simulink model "different_inverter_controls_BPS"  (R2024b)
settings: Solver=ode4  StartTime=0.0  StopTime=5  FixedStep=Ts  RelTol=1e-3
InitFcn:
  | %mode_of_operation=1;
  | %BESS_control_mode=1;
  | %Gen_Q_Control =1;
  | 
  | %Exciter_init;
  | 
  | %Exciter_init
  | Xq=0.474;
  | %%====================================================
  | % ST6C Exciter Parameters
  | 
  | KPA=30;
  | KIA=59.91;
  | KFF=1;
  | KM=1;
  | KLR=22.47;
  | KCL=1.04;
  | VAMAX=7.05;
  | VAMIN=-6.11;
  | VRMAX=7.05;
  | VRMIN=-6.11;
  | ILR=5.02;
  | KG=1;
  | TG=0.024;
  | TA=0.01;
  | VBMAX=999;
  | VMMAX=7.05;
  | VMMIN=-6.11;
  | KI=0;
  | Kp=1;
  | Kc=0;
  | Vt0=0;
  | VAAMAX=VAMAX;
  | %%========================================================
  | % UEL2C parameters
  | 
  | TUQ=.005;
  | TUP=0.050;
  | TUV=0.2;
  | TQREF=0;
  | Tadj=0;
  | K1=0;
  | K2=2;
  | VBIAS=1;
  | KFB=0;
  | TUL=0;
  | VUImax=1;
  | VUImin=-1;
  | VUELmax1=1;
  | VUELmax2=1;
  | VUELmin1=-1;
  | VUELmin2=-1;
  | KUF=0;
  | KUL=0.24;
  | KUI=0.001;
  | TU1=0;TU2=0;TU3=0;TU4=0;
  | KFIX=1;
  | VF=0;
  | VFB=0;
  | %%===========================================================
  | ... (+60 lines)
values from neighbouring files (symbols this model uses):
  inv1 = struct    [multiInverterParams.m]
  kp_sync = KQ_p/10    (= 0.04)    [multiInverterParams.m]
  Vdc = 1000    [multiInverterParams.m]
  Vpp = 480    [multiInverterParams.m]
undefined symbols (not defined in the file or in its folder): D1, Delta, DiscIntNeverNeededParam, Ion, Lithium, sigbuilder_block, sps
libraries: slpidlib x34, spsThreePhaseVIMeasurementLib x31, spsThreePhaseSeriesRLCBranchLib x23, spsabctodq0Lib x22, spsPower3phInstantaneousLib x22, spsThreePhaseTransformerTwoWindingsLib x16, spsSeriesRLCBranchLib x16, spsThreePhaseSeriesRLCLoadLib x14, simulink x12, spsPLL3phLib x11, spsGroundLib x9, powerlib_extras x8
(part 6 of 9)

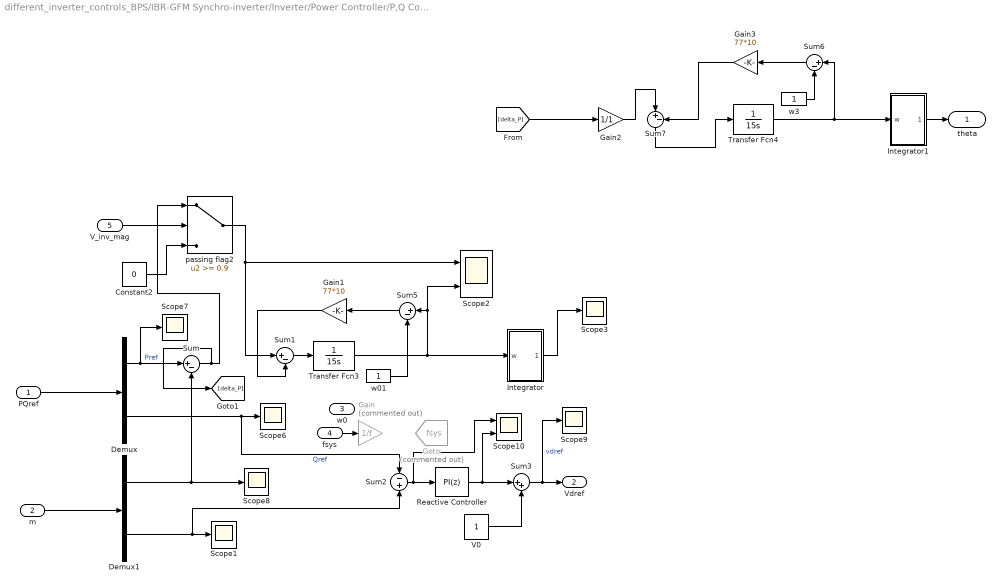
== system different_inverter_controls_BPS/IBR-GFM Synchro-inverter/Inverter/Power Controller/P,Q Control  ==
  PQref : Inport
  m : Inport  Port=2
  w0 : Inport  Port=3
  fsys : Inport  Port=4
  V_inv_mag : Inport  Port=5
  Constant2 : Constant  Value=0  SampleTime=Ts_Control
  Demux : Demux  Outputs=2
  Demux1 : Demux  Outputs=2
  Gain : Gain  Commented=on  Gain=1/f
  Gain1 : Gain  Gain=77*10
  Gain2 : Gain  Gain=1/1
  Gain3 : Gain  Gain=77*10
  Goto : Goto  Commented=on  GotoTag=fsys  TagVisibility=global
  Integrator : Subsystem
  Integrator1 : Subsystem
  Reactive Controller : slpidlib/PID Controller  Controller=PI  Form=Parallel  TimeDomain=Discrete-time  UseExternalTs=off  SampleTime=Ts_Control  IntegratorMethod=Forward Euler  FilterMethod=Forward Euler  ControllerParametersSource=internal  P=-.001  I=0  UseKiTs=off  D=0  UseExternalDerivativeSource=off  N=100  UseFilter=on  TunerSelectOption=Transfer Function Based (PID Tuner App)  InitialConditionSource=internal  InitialConditionForIntegrator=0  InitialConditionForFilter=0  DifferentiatorICPrevScaledInput=0  ExternalReset=none  TrackingMode=off  Kt=1  LimitOutput=on  SatLimitsSource=internal  UpperSaturationLimit=1.5  LowerSaturationLimit=-1.5  LinearizeAsGain=off  AntiWindupMode=back-calculation  Kb=1  LimitIntegrator=off  UpperIntegratorSaturationLimit=inf  LowerIntegratorSaturationLimit=-inf  POutMin=[]  POutMax=[]  IOutMin=[]  IOutMax=[]  DOutMin=[]  DOutMax=[]  NOutMin=[]  NOutMax=[]  SumOutMin=[]  SumOutMax=[]  SaturationOutMin=[]  SaturationOutMax=[]  PParamMin=[]  PParamMax=[]  IParamMin=[]  IParamMax=[]  DParamMin=[]  DParamMax=[]  NParamMin=[]  NParamMax=[]  KbParamMin=[]  KbParamMax=[]  KtParamMin=[]  KtParamMax=[]  KbOutMin=[]  KbOutMax=[]  KtOutMin=[]  KtOutMax=[]  IntegratorOutMin=[]  IntegratorOutMax=[]  FilterOutMin=[]  FilterOutMax=[]  SumI1OutMin=[]  SumI1OutMax=[]  SumI2OutMin=[]  SumI2OutMax=[]  SumI3OutMin=[]  SumI3OutMax=[]  SumI4OutMin=[]  SumI4OutMax=[]  SumDOutMin=[]  SumDOutMax=[]  DifferentiatorOutMin=[]  DifferentiatorOutMax=[]  FilterDiffOutCoefMin=[]  FilterDiffOutCoefMax=[]  ReciprocalOutMin=[]  ReciprocalOutMax=[]  SumDenOutMin=[]  SumDenOutMax=[]  SumNumOutMin=[]  SumNumOutMax=[]  DivideOutMin=[]  DivideOutMax=[]  UdiffTsProdOutMin=[]  UdiffTsProdOutMax=[]  NTsProdOutMin=[]  NTsProdOutMax=[]  UintegralTsProdOutMin=[]  UintegralTsProdOutMax=[]  UngainTsProdOutMin=[]  UngainTsProdOutMax=[]  ClampingZeroOutDataTypeStr=Inherit: Inherit via back propagation  ClampingZeroOutMin=[]  ClampingZeroOutMax=[]  FilterDenConstantOutDataTypeStr=Inherit: Inherit via back propagation  FilterDenConstantOutMin=[]  FilterDenConstantOutMax=[]  PCopyOutDataTypeStr=Inherit: Inherit via back propagation  PCopyOutMin=[]  PCopyOutMax=[]  NCopyOutDataTypeStr=Inherit: Inherit via back propagation  NCopyOutMin=[]  NCopyOutMax=[]  IntegratorContinuousStateAttributes=''  IntegratorStateMustResolveToSignalObject=off  IntegratorRTWStateStorageClass=Auto  FilterContinuousStateAttributes=''  FilterStateMustResolveToSignalObject=off  FilterRTWStateStorageClass=Auto  ParallelPVariant=InternalParameters  IdealPVariant=Disabled  IVariant=InternalParameters  DVariant=Disabled  IntegratorVariant=Discrete  SatVariant=Enabled  AWVariant=BackCalculation  PCopyVariant=Disabled  TRVariant=Disabled  FdbkBlocksVariant=Forward  IdealPFdbkVariant=Disabled  SatFdbkVariant=Disabled  DerivativeFilterVariant=Disabled  NVariant=Disabled  NCopyVariant=Disabled_SignalSpec  FilterICVariant=Disabled  IntegratorICVariant=InternalICs  ExternalResetVariant=Disabled  TRSumVariant=Passthrough  SumFdbkVariant=Disabled  SumVariant=Sum_PI  TsampFilterVariant=InternalTs  TsampNgainVariant=Passthrough  TsampIntegralVariant=Disabled_SignalSpec  ExternalSaturationOutDataTypeStr=Inherit: Same as second input  DerivativeSourceVariant=Disabled  PreIntVariant=InternalPreInt
  Scope{1,3,6..9} (6 alike) : Scope
  Scope10 : Scope  NumInputPorts=2
  Scope2 : Scope  NumInputPorts=2
  Sum{,1,5..7} (5 alike) : Sum  Inputs=|+-
  Sum2 : Sum  Inputs=-+
  Sum3 : Sum  Inputs=|++
  Transfer Fcn3 : TransferFcn  Denominator=[15 0]
  Transfer Fcn4 : TransferFcn  Denominator=[15 0]
  V0 : Constant  SampleTime=Ts_Control
  passing flag2 : Switch  Threshold=0.9  SaturateOnIntegerOverflow=off  InputSameDT=off
  w01 : Constant  SampleTime=Ts_Control
  w3 : Constant  SampleTime=Ts_Control
  theta : Outport  VectorParamsAs1DForOutWhenUnconnected=off
  Vdref : Outport  Port=2
  wires:
  Integrator1/1(Theta) -> theta/1
  w3/1 -> Sum6/2
  Transfer Fcn4/1 -> Sum6/1, Integrator1/1(w)
  Sum7/1 -> Transfer Fcn4/1
  Gain3/1 -> Sum7/2
  Gain2/1 -> Sum7/1
  Sum6/1 -> Gain3/1
  [delta_P] -> Gain2/1
  w01/1 -> Sum5/2
  passing flag2/1 -> Scope2/1, Sum1/1
  Sum/1 -> passing flag2/1, [delta_P]
  Transfer Fcn3/1 -> Sum5/1, Scope2/2, Integrator/1(w)
  Sum1/1 -> Transfer Fcn3/1
  Gain1/1 -> Sum1/2
  Sum5/1 -> Gain1/1
  fsys/1 -> Gain/1
  Constant2/1 -> passing flag2/3
  V_inv_mag/1 -> passing flag2/2
  Sum3/1 -> Vdref/1, Scope9/1  "vdref"
  V0/1 -> Sum3/2
  Reactive Controller/1 -> Sum3/1, Scope10/2
  Sum2/1 -> Reactive Controller/1, Scope10/1
  Demux1/2 -> Scope1/1, Sum2/2
  Demux/2 -> Scope6/1, Sum2/1  "Qref"
  Demux/1 -> Sum/1, Scope7/1  "Pref"
  PQref/1 -> Demux/1
  m/1 -> Demux1/1
  Demux1/1 -> Scope8/1, Sum/2
  Integrator/1(Theta) -> Scope3/1

== system different_inverter_controls_BPS/IBR-GFM Power Synchronization/Inverter/ Reference /Qref ==
  Constant : Constant  Value=44e6
  From1 : From  Commented=on  GotoTag=Q_BESS
  Out1 : Outport
  wires:
  Constant/1 -> Out1/1

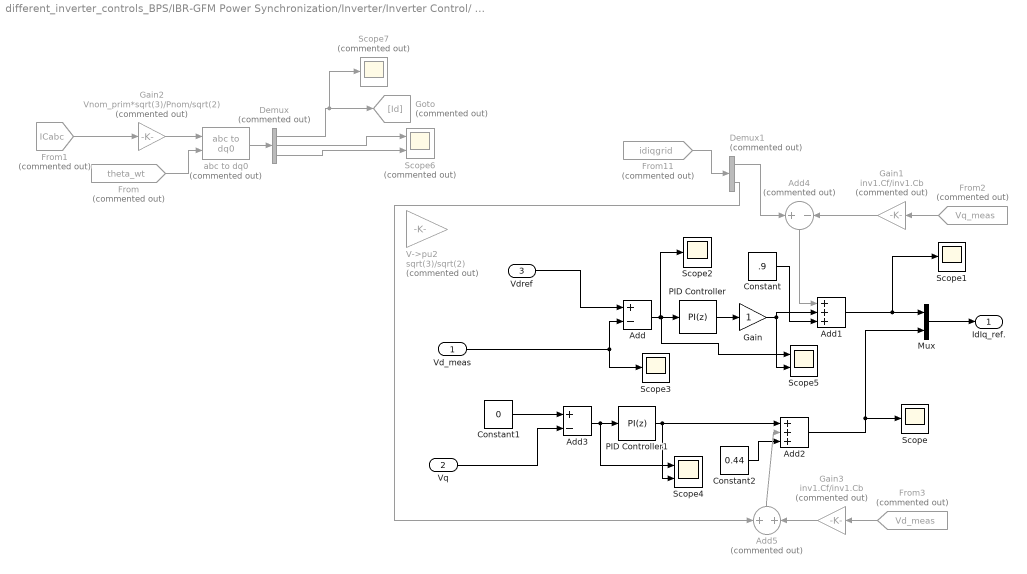
== system different_inverter_controls_BPS/IBR-GFM Power Synchronization/Inverter/Inverter Control/ voltage control  ==
  Vd_meas : Inport
  Vq : Inport  Port=2
  Vdref : Inport  Port=3
  Add : Sum  Inputs=+-
  Add1 : Sum  Inputs=+++
  Add2 : Sum  Inputs=+++
  Add3 : Sum  Inputs=+-
  Add4 : Sum  Commented=on  Inputs=+-
  Add5 : Sum  Commented=on
  Constant : Constant  Value=.9  SampleTime=Ts_Control
  Constant1 : Constant  Value=0
  Constant2 : Constant  Value=0.44
  Demux : Demux  Commented=on  Outputs=3
  Demux1 : Demux  Commented=on  Outputs=2
  From : From  Commented=on  GotoTag=theta_wt  TagVisibility=global
  From1 : From  Commented=on  GotoTag=ICabc  TagVisibility=global
  From11 : From  Commented=on  GotoTag=idiqgrid  TagVisibility=global
  From2 : From  Commented=on  GotoTag=Vq_meas  TagVisibility=global
  From3 : From  Commented=on  GotoTag=Vd_meas  TagVisibility=global
  Gain : Gain
  Gain1 : Gain  Commented=on  Gain=inv1.Cf/inv1.Cb
  Gain2 : Gain  Commented=on  Gain=Vnom_prim*sqrt(3)/Pnom/sqrt(2)
  Gain3 : Gain  Commented=on  Gain=inv1.Cf/inv1.Cb
  Goto : Goto  Commented=on  GotoTag=Id
  Mux : Mux  Inputs=2
  PID Controller : slpidlib/PID Controller  Controller=PI  Form=Parallel  TimeDomain=Discrete-time  UseExternalTs=off  SampleTime=Ts_Control  IntegratorMethod=Forward Euler  FilterMethod=Forward Euler  ControllerParametersSource=internal  P=.8  I=0  D=0  UseFilter=on  N=100  TunerSelectOption=Transfer Function Based (PID Tuner App)  InitialConditionSource=internal  InitialConditionForIntegrator=0  InitialConditionForFilter=0  DifferentiatorICPrevScaledInput=0  ExternalReset=none  TrackingMode=off  Kt=1  LimitOutput=on  SatLimitsSource=internal  UpperSaturationLimit=inf  LowerSaturationLimit=-inf  LinearizeAsGain=on  AntiWindupMode=back-calculation  Kb=1  POutMin=[]  POutMax=[]  IOutMin=[]  IOutMax=[]  DOutMin=[]  DOutMax=[]  NOutMin=[]  NOutMax=[]  SumOutMin=[]  SumOutMax=[]  SaturationOutMin=[]  SaturationOutMax=[]  PParamMin=[]  PParamMax=[]  IParamMin=[]  IParamMax=[]  DParamMin=[]  DParamMax=[]  NParamMin=[]  NParamMax=[]  KbParamMin=[]  KbParamMax=[]  KtParamMin=[]  KtParamMax=[]  KbOutMin=[]  KbOutMax=[]  KtOutMin=[]  KtOutMax=[]  IntegratorOutMin=[]  IntegratorOutMax=[]  FilterOutMin=[]  FilterOutMax=[]  SumI1OutMin=[]  SumI1OutMax=[]  SumI2OutMin=[]  SumI2OutMax=[]  SumI3OutMin=[]  SumI3OutMax=[]  SumI4OutMin=[]  SumI4OutMax=[]  SumDOutMin=[]  SumDOutMax=[]  DifferentiatorOutMin=[]  DifferentiatorOutMax=[]  FilterDiffOutCoefMin=[]  FilterDiffOutCoefMax=[]  ReciprocalOutMin=[]  ReciprocalOutMax=[]  SumDenOutMin=[]  SumDenOutMax=[]  SumNumOutMin=[]  SumNumOutMax=[]  DivideOutMin=[]  DivideOutMax=[]  UdiffTsProdOutMin=[]  UdiffTsProdOutMax=[]  NTsProdOutMin=[]  NTsProdOutMax=[]  UintegralTsProdOutMin=[]  UintegralTsProdOutMax=[]  UngainTsProdOutMin=[]  UngainTsProdOutMax=[]  FilterDenConstantOutDataTypeStr=Inherit: Inherit via back propagation  FilterDenConstantOutMin=[]  FilterDenConstantOutMax=[]  PCopyOutDataTypeStr=Inherit: Inherit via back propagation  PCopyOutMin=[]  PCopyOutMax=[]  NCopyOutDataTypeStr=Inherit: Inherit via back propagation  NCopyOutMin=[]  NCopyOutMax=[]  IntegratorContinuousStateAttributes=''  IntegratorStateMustResolveToSignalObject=off  IntegratorRTWStateStorageClass=Auto  FilterContinuousStateAttributes=''  FilterStateMustResolveToSignalObject=off  FilterRTWStateStorageClass=Auto  ParallelPVariant=InternalParameters  IdealPVariant=Disabled  IVariant=InternalParameters  DVariant=Disabled  IntegratorVariant=Discrete  SatVariant=Enabled  AWVariant=BackCalculation  PCopyVariant=Disabled  TRVariant=Disabled  FdbkBlocksVariant=Forward  IdealPFdbkVariant=Disabled  SatFdbkVariant=Disabled  DerivativeFilterVariant=Disabled  NVariant=Disabled  NCopyVariant=Disabled_SignalSpec  FilterICVariant=Disabled  IntegratorICVariant=InternalICs  ExternalResetVariant=Disabled  TRSumVariant=Passthrough  SumFdbkVariant=Disabled  SumVariant=Sum_PI  TsampFilterVariant=InternalTs  TsampNgainVariant=Passthrough  TsampIntegralVariant=Passthrough  ExternalSaturationOutDataTypeStr=Inherit: Same as second input
  PID Controller1 : slpidlib/PID Controller  Controller=PI  Form=Parallel  TimeDomain=Discrete-time  UseExternalTs=off  SampleTime=Ts_Control  IntegratorMethod=Forward Euler  FilterMethod=Forward Euler  ControllerParametersSource=internal  P=.79  I=0  D=0  UseFilter=on  N=100  TunerSelectOption=Transfer Function Based (PID Tuner App)  InitialConditionSource=internal  InitialConditionForIntegrator=0  InitialConditionForFilter=0  DifferentiatorICPrevScaledInput=0  ExternalReset=none  TrackingMode=off  Kt=1  LimitOutput=on  SatLimitsSource=internal  UpperSaturationLimit=inf  LowerSaturationLimit=-inf  LinearizeAsGain=on  AntiWindupMode=back-calculation  Kb=1  POutMin=[]  POutMax=[]  IOutMin=[]  IOutMax=[]  DOutMin=[]  DOutMax=[]  NOutMin=[]  NOutMax=[]  SumOutMin=[]  SumOutMax=[]  SaturationOutMin=[]  SaturationOutMax=[]  PParamMin=[]  PParamMax=[]  IParamMin=[]  IParamMax=[]  DParamMin=[]  DParamMax=[]  NParamMin=[]  NParamMax=[]  KbParamMin=[]  KbParamMax=[]  KtParamMin=[]  KtParamMax=[]  KbOutMin=[]  KbOutMax=[]  KtOutMin=[]  KtOutMax=[]  IntegratorOutMin=[]  IntegratorOutMax=[]  FilterOutMin=[]  FilterOutMax=[]  SumI1OutMin=[]  SumI1OutMax=[]  SumI2OutMin=[]  SumI2OutMax=[]  SumI3OutMin=[]  SumI3OutMax=[]  SumI4OutMin=[]  SumI4OutMax=[]  SumDOutMin=[]  SumDOutMax=[]  DifferentiatorOutMin=[]  DifferentiatorOutMax=[]  FilterDiffOutCoefMin=[]  FilterDiffOutCoefMax=[]  ReciprocalOutMin=[]  ReciprocalOutMax=[]  SumDenOutMin=[]  SumDenOutMax=[]  SumNumOutMin=[]  SumNumOutMax=[]  DivideOutMin=[]  DivideOutMax=[]  UdiffTsProdOutMin=[]  UdiffTsProdOutMax=[]  NTsProdOutMin=[]  NTsProdOutMax=[]  UintegralTsProdOutMin=[]  UintegralTsProdOutMax=[]  UngainTsProdOutMin=[]  UngainTsProdOutMax=[]  FilterDenConstantOutDataTypeStr=Inherit: Inherit via back propagation  FilterDenConstantOutMin=[]  FilterDenConstantOutMax=[]  PCopyOutDataTypeStr=Inherit: Inherit via back propagation  PCopyOutMin=[]  PCopyOutMax=[]  NCopyOutDataTypeStr=Inherit: Inherit via back propagation  NCopyOutMin=[]  NCopyOutMax=[]  IntegratorContinuousStateAttributes=''  IntegratorStateMustResolveToSignalObject=off  IntegratorRTWStateStorageClass=Auto  FilterContinuousStateAttributes=''  FilterStateMustResolveToSignalObject=off  FilterRTWStateStorageClass=Auto  ParallelPVariant=InternalParameters  IdealPVariant=Disabled  IVariant=InternalParameters  DVariant=Disabled  IntegratorVariant=Discrete  SatVariant=Enabled  AWVariant=BackCalculation  PCopyVariant=Disabled  TRVariant=Disabled  FdbkBlocksVariant=Forward  IdealPFdbkVariant=Disabled  SatFdbkVariant=Disabled  DerivativeFilterVariant=Disabled  NVariant=Disabled  NCopyVariant=Disabled_SignalSpec  FilterICVariant=Disabled  IntegratorICVariant=InternalICs  ExternalResetVariant=Disabled  TRSumVariant=Passthrough  SumFdbkVariant=Disabled  SumVariant=Sum_PI  TsampFilterVariant=InternalTs  TsampNgainVariant=Passthrough  TsampIntegralVariant=Passthrough  ExternalSaturationOutDataTypeStr=Inherit: Same as second input
  Scope{,1..3} (4 alike) : Scope
  Scope4 : Scope  NumInputPorts=2
  Scope5 : Scope  NumInputPorts=2
  Scope6 : Scope  Commented=on  NumInputPorts=2
  Scope7 : Scope  Commented=on
  V->pu2 : Gain  Commented=on  Gain=sqrt(3)/sqrt(2)  SaturateOnIntegerOverflow=on  OutDataTypeStr=Inherit: Same as input  ParamDataTypeStr=Inherit: Same as input
  abc to dq0 : spsabctodq0Lib/abc to dq0  Commented=on  Alignment=90 degrees behind phase A axis
  IdIq_ref. : Outport
  wires:
  Constant2/1 -> Add2/3
  Constant/1 -> Add1/3
  From3/1 -> Gain3/1
  Gain3/1 -> Add5/2
  Add5/1 -> Add2/2
  Demux1/2 -> Add5/1
  From2/1 -> Gain1/1
  Gain1/1 -> Add4/2
  Demux1/1 -> Add4/1
  From11/1 -> Demux1/1
  Add4/1 -> Add1/1
  Add3/1 -> PID Controller1/1, Scope4/1
  Vq/1 -> Add3/2
  Constant1/1 -> Add3/1
  Vdref/1 -> Add/1
  Vd_meas/1 -> Add/2, Scope3/1
  PID Controller/1 -> Gain/1
  Add/1 -> Scope2/1, PID Controller/1, Scope5/1
  Mux/1 -> IdIq_ref./1
  Gain/1 -> Scope5/2, Add1/2
  Add1/1 -> Scope1/1, Mux/1
  PID Controller1/1 -> Scope4/2, Add2/1
  Add2/1 -> Scope/1, Mux/2
  From/1 -> abc to dq0/2
  Gain2/1 -> abc to dq0/1
  From1/1 -> Gain2/1
  abc to dq0/1 -> Demux/1
  Demux/1 -> Scope7/1, Goto/1
  Demux/2 -> Scope6/1
  Demux/3 -> Scope6/2

== system different_inverter_controls_BPS/IBR-GFM Power Synchronization/Inverter/Inverter Control/Conversions ==
  Vabc_prim : Inport
  Iabc_prim : Inport  Port=2
  Iabc_grid : Inport  Port=3
  From1 : From  Commented=on  GotoTag=theta_inv  TagVisibility=global
  From2 : From  Commented=on  GotoTag=theta  TagVisibility=global
  Goto7 : Goto  Commented=on  GotoTag=theta_inv  TagVisibility=global
  PLL (3ph)1 : spsPLL3phLib/PLL (3ph)  Fmin=45  Par_Init="[-0.57  Fnom]"  ParK=[180, 3200, 1]  TcD=1e-04  MaxRateChangeFreq=12  FilterCutOffFreq=25  Ts=Ts_Control  AGC=on
      link override Model/Constant4: Value=2*pi
  "PMU (PLL-Based, Positive-Sequence)" : spsPMUPLLBasedPositiveSequenceLib/PMU (PLL-Based, Positive-Sequence)  Commented=on  nominalFrequency=50  samplingRate=64  reportingFactor=1
  Scope{,1..3,7} (5 alike) : Scope
  Scope4 : Scope  Commented=on
  Scope5 : Scope  Commented=on
  Scope6 : Scope  Commented=on
  Selector1 : Selector  InputPortWidth=3  IndexOptions=Index vector (dialog)  Indices=[1 2]  OutputSizes=1
  Selector2 : Selector  InputPortWidth=3  IndexOptions=Index vector (dialog)  Indices=[1 2]  OutputSizes=1
  Selector3 : Selector  Commented=on  InputPortWidth=3  IndexOptions=Index vector (dialog)  Indices=[1 2]  OutputSizes=1
  Terminator : Terminator  Commented=on
  Terminator1 : Terminator  Commented=on
  V->pu : Gain  Gain=1/(Vpp*sqrt(2)/sqrt(3))  SaturateOnIntegerOverflow=on  OutDataTypeStr=Inherit: Same as input  ParamDataTypeStr=Inherit: Same as input
  V->pu1 : Gain  Gain=Vpp*sqrt(3)/Pnom/sqrt(2)  SaturateOnIntegerOverflow=on  OutDataTypeStr=Inherit: Same as input  ParamDataTypeStr=Inherit: Same as input
  V->pu2 : Gain  Commented=on  Gain=1/(Vnom_prim*sqrt(2)/sqrt(3))  SaturateOnIntegerOverflow=on  OutDataTypeStr=Inherit: Same as input  ParamDataTypeStr=Inherit: Same as input
  V->pu3 : Gain  Commented=on  Gain=Vnom_prim*sqrt(3)/Pnom/sqrt(2)  SaturateOnIntegerOverflow=on  OutDataTypeStr=Inherit: Same as input  ParamDataTypeStr=Inherit: Same as input
  V->pu4 : Gain  Commented=on  Gain=1/(Vpp*sqrt(2)/sqrt(3))  SaturateOnIntegerOverflow=on  OutDataTypeStr=Inherit: Same as input  ParamDataTypeStr=Inherit: Same as input
  V->pu6 : Gain  Commented=on  Gain=Vnom_prim*sqrt(3)/Pnom/sqrt(2)  SaturateOnIntegerOverflow=on  OutDataTypeStr=Inherit: Same as input  ParamDataTypeStr=Inherit: Same as input
  abc to dq0 : spsabctodq0Lib/abc to dq0  Alignment=90 degrees behind phase A axis
  abc to dq1 : spsabctodq0Lib/abc to dq0  Alignment=90 degrees behind phase A axis
  abc to dq2 : spsabctodq0Lib/abc to dq0  Commented=on  Alignment=90 degrees behind phase A axis
  wt : Outport  VectorParamsAs1DForOutWhenUnconnected=off
  VdVq_prim : Outport  Port=2  VectorParamsAs1DForOutWhenUnconnected=off
  IdIq_prim : Outport  Port=3  VectorParamsAs1DForOutWhenUnconnected=off
  IdIq_grid : Outport  Port=4  VectorParamsAs1DForOutWhenUnconnected=off
  tag scope: PLL_Freq=scoped, theta_wt=global
  wires:
  Iabc_grid/1 -> abc to dq2/1, Scope5/1
  Selector3/1 -> IdIq_grid/1, Scope6/1
  abc to dq2/1 -> Selector3/1
  [theta] -> abc to dq1/2, abc to dq2/2, abc to dq0/2
  "PMU (PLL-Based, Positive-Sequence)"/1 -> Terminator1/1
  "PMU (PLL-Based, Positive-Sequence)"/3 -> Terminator/1
  "PMU (PLL-Based, Positive-Sequence)"/2 -> Goto7/1, Scope4/1
  PLL (3ph)1/1 -> [PLL_Freq], Scope3/1
  V->pu/1 -> abc to dq0/1, Scope7/1, PLL (3ph)1/1, "PMU (PLL-Based, Positive-Sequence)"/1
  abc to dq1/1 -> Selector1/1
  Vabc_prim/1 -> V->pu/1
  Iabc_prim/1 -> V->pu1/1
  abc to dq0/1 -> Selector2/1
  Selector2/1 -> VdVq_prim/1
  Selector1/1 -> Scope2/1, IdIq_prim/1
  PLL (3ph)1/2 -> wt/1, [theta_wt], Scope/1
  V->pu1/1 -> Scope1/1, abc to dq1/1

== system different_inverter_controls_BPS/IBR-GFM Power Synchronization/Inverter/Inverter Control/Current Control ==
  wt : Inport
  VdVq_meas : Inport  Port=2  PortDimensions=2
  IdIq_meas : Inport  Port=3  PortDimensions=2
  IdIq_ref : Inport  Port=4  PortDimensions=2
  Current Regulator : Subsystem
  Uabc_ref Generation max (m) = 1 : Subsystem
  Uabc : Outport  VectorParamsAs1DForOutWhenUnconnected=off
  wires:
  Uabc_ref Generation max (m) = 1/1(Uabc_ref) -> Uabc/1
  IdIq_ref/1 -> Current Regulator/3(IdIq_ref)
  IdIq_meas/1 -> Current Regulator/2(IdIq_meas)
  VdVq_meas/1 -> Current Regulator/1(VdVq_meas)
  Current Regulator/1(VdVq_conv) -> Uabc_ref Generation max (m) = 1/2(VdVq_conv)
  wt/1 -> Uabc_ref Generation max (m) = 1/1(wt)

== system different_inverter_controls_BPS/IBR-GFM Power Synchronization/Inverter/Inverter Control/current limiter ==
  note: P or Q priority limits are usually applied during grid feeding mode of operation
      | https://www.esig.energy/wiki-main-page/wecc-distributed-and-small-pv-plants-generic-model-pvd1/
  idiqPref : Inport
  V_inv_mag : Inport  Port=2
  P priority limit : Subsystem  Commented=on
  Q priority limit : Subsystem
  Subsystem3 : Subsystem  Commented=on
  Subsystem4 : Subsystem  Commented=on
  Subsystem9 : Subsystem
  Switch1 : Switch  Commented=on  Criteria=u2 > Threshold  SaturateOnIntegerOverflow=off  InputSameDT=off
  idiqPRefL : Outport
  wires:
  V_inv_mag/1 -> Q priority limit/2(V_inv_mag)
  [mode] -> Switch1/2
  Q priority limit/1(idiqPRefL) -> Switch1/3, idiqPRefL/1
  idiqPref/1 -> Subsystem4/2(In2), Subsystem9/2(In2), Q priority limit/1(idiqP), P priority limit/1(idiqP), Subsystem3/1(In1)
  Subsystem3/1(Out1) -> [Ivector]
  [Ivector] -> Subsystem4/1(In1)
  Subsystem4/1(Out1) -> Switch1/1
  [Ivector] -> Subsystem9/1(In1)
  Subsystem3/2(Out2) -> [IPvector]

== system different_inverter_controls_BPS/IBR-GFM Power Synchronization/Inverter/Power Controller/Compute PQ ==
  m : Inport
  Bus Selector : BusSelector  OutputSignals=Vabc,Iabc
  Mux : Mux  Inputs=2
  "Power (3ph, Instantaneous)" : spsPower3phInstantaneousLib/Power (3ph, Instantaneous)
  Scope1 : Scope
  to PU : Gain  Gain=1/Pnom
  "to PU " : Gain  Gain=1/Pnom
  to PU1 : Gain  Commented=on  Gain=1/Pnom
  PQm : Outport  VectorParamsAs1DForOutWhenUnconnected=off
  wires:
  Bus Selector/1 -> "Power (3ph, Instantaneous)"/1  "<Vabc>"
  "Power (3ph, Instantaneous)"/2 -> "to PU "/1
  Bus Selector/2 -> "Power (3ph, Instantaneous)"/2  "<Iabc>"
  "Power (3ph, Instantaneous)"/1 -> to PU/1
  m/1 -> Bus Selector/1
  to PU/1 -> Mux/1
  "to PU "/1 -> Mux/2
  Mux/1 -> PQm/1, Scope1/1

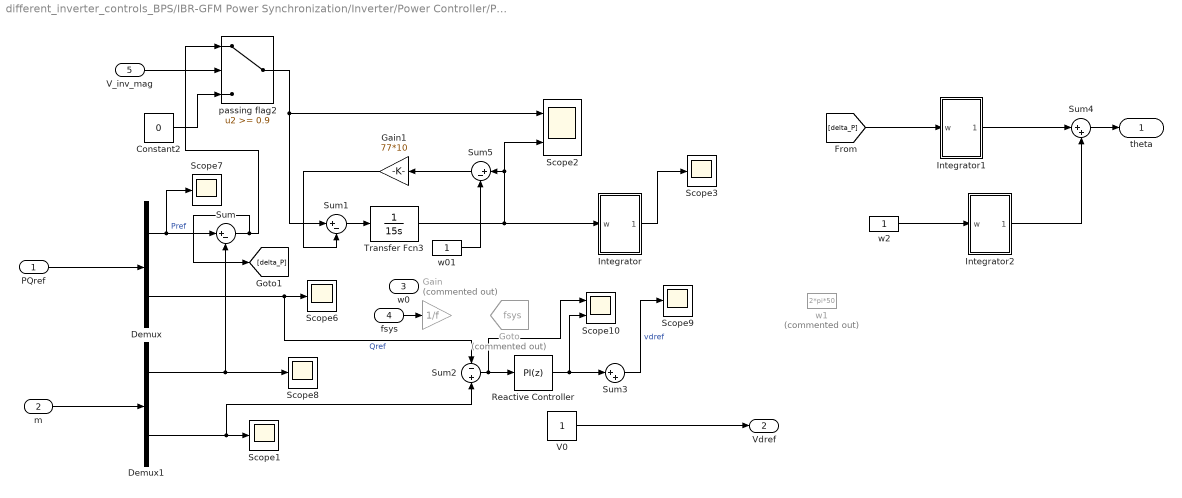
== system different_inverter_controls_BPS/IBR-GFM Power Synchronization/Inverter/Power Controller/P,Q Control  ==
  PQref : Inport
  m : Inport  Port=2
  w0 : Inport  Port=3
  fsys : Inport  Port=4
  V_inv_mag : Inport  Port=5
  Constant2 : Constant  Value=0  SampleTime=Ts_Control
  Demux : Demux  Outputs=2
  Demux1 : Demux  Outputs=2
  Gain : Gain  Commented=on  Gain=1/f
  Gain1 : Gain  Gain=77*10
  Goto : Goto  Commented=on  GotoTag=fsys  TagVisibility=global
  Integrator : Subsystem
  Integrator1 : Subsystem
  Integrator2 : Subsystem
  Reactive Controller : slpidlib/PID Controller  Controller=PI  Form=Parallel  TimeDomain=Discrete-time  UseExternalTs=off  SampleTime=Ts_Control  IntegratorMethod=Forward Euler  FilterMethod=Forward Euler  ControllerParametersSource=internal  P=-.001  I=0  UseKiTs=off  D=0  UseExternalDerivativeSource=off  N=100  UseFilter=on  TunerSelectOption=Transfer Function Based (PID Tuner App)  InitialConditionSource=internal  InitialConditionForIntegrator=0  InitialConditionForFilter=0  DifferentiatorICPrevScaledInput=0  ExternalReset=none  TrackingMode=off  Kt=1  LimitOutput=on  SatLimitsSource=internal  UpperSaturationLimit=1.5  LowerSaturationLimit=-1.5  LinearizeAsGain=off  AntiWindupMode=back-calculation  Kb=1  LimitIntegrator=off  UpperIntegratorSaturationLimit=inf  LowerIntegratorSaturationLimit=-inf  POutMin=[]  POutMax=[]  IOutMin=[]  IOutMax=[]  DOutMin=[]  DOutMax=[]  NOutMin=[]  NOutMax=[]  SumOutMin=[]  SumOutMax=[]  SaturationOutMin=[]  SaturationOutMax=[]  PParamMin=[]  PParamMax=[]  IParamMin=[]  IParamMax=[]  DParamMin=[]  DParamMax=[]  NParamMin=[]  NParamMax=[]  KbParamMin=[]  KbParamMax=[]  KtParamMin=[]  KtParamMax=[]  KbOutMin=[]  KbOutMax=[]  KtOutMin=[]  KtOutMax=[]  IntegratorOutMin=[]  IntegratorOutMax=[]  FilterOutMin=[]  FilterOutMax=[]  SumI1OutMin=[]  SumI1OutMax=[]  SumI2OutMin=[]  SumI2OutMax=[]  SumI3OutMin=[]  SumI3OutMax=[]  SumI4OutMin=[]  SumI4OutMax=[]  SumDOutMin=[]  SumDOutMax=[]  DifferentiatorOutMin=[]  DifferentiatorOutMax=[]  FilterDiffOutCoefMin=[]  FilterDiffOutCoefMax=[]  ReciprocalOutMin=[]  ReciprocalOutMax=[]  SumDenOutMin=[]  SumDenOutMax=[]  SumNumOutMin=[]  SumNumOutMax=[]  DivideOutMin=[]  DivideOutMax=[]  UdiffTsProdOutMin=[]  UdiffTsProdOutMax=[]  NTsProdOutMin=[]  NTsProdOutMax=[]  UintegralTsProdOutMin=[]  UintegralTsProdOutMax=[]  UngainTsProdOutMin=[]  UngainTsProdOutMax=[]  ClampingZeroOutDataTypeStr=Inherit: Inherit via back propagation  ClampingZeroOutMin=[]  ClampingZeroOutMax=[]  FilterDenConstantOutDataTypeStr=Inherit: Inherit via back propagation  FilterDenConstantOutMin=[]  FilterDenConstantOutMax=[]  PCopyOutDataTypeStr=Inherit: Inherit via back propagation  PCopyOutMin=[]  PCopyOutMax=[]  NCopyOutDataTypeStr=Inherit: Inherit via back propagation  NCopyOutMin=[]  NCopyOutMax=[]  IntegratorContinuousStateAttributes=''  IntegratorStateMustResolveToSignalObject=off  IntegratorRTWStateStorageClass=Auto  FilterContinuousStateAttributes=''  FilterStateMustResolveToSignalObject=off  FilterRTWStateStorageClass=Auto  ParallelPVariant=InternalParameters  IdealPVariant=Disabled  IVariant=InternalParameters  DVariant=Disabled  IntegratorVariant=Discrete  SatVariant=Enabled  AWVariant=BackCalculation  PCopyVariant=Disabled  TRVariant=Disabled  FdbkBlocksVariant=Forward  IdealPFdbkVariant=Disabled  SatFdbkVariant=Disabled  DerivativeFilterVariant=Disabled  NVariant=Disabled  NCopyVariant=Disabled_SignalSpec  FilterICVariant=Disabled  IntegratorICVariant=InternalICs  ExternalResetVariant=Disabled  TRSumVariant=Passthrough  SumFdbkVariant=Disabled  SumVariant=Sum_PI  TsampFilterVariant=InternalTs  TsampNgainVariant=Passthrough  TsampIntegralVariant=Disabled_SignalSpec  ExternalSaturationOutDataTypeStr=Inherit: Same as second input  DerivativeSourceVariant=Disabled  PreIntVariant=InternalPreInt
  Scope{1,3,6..9} (6 alike) : Scope
  Scope10 : Scope  NumInputPorts=2
  Scope2 : Scope  NumInputPorts=2
  Sum : Sum  Inputs=|+-
  Sum1 : Sum  Inputs=|+-
  Sum2 : Sum  Inputs=-+
  Sum3 : Sum  Inputs=|++
  Sum4 : Sum  Inputs=|++
  Sum5 : Sum  Inputs=|+-
  Transfer Fcn3 : TransferFcn  Denominator=[15 0]
  V0 : Constant  SampleTime=Ts_Control
  passing flag2 : Switch  Threshold=0.9  SaturateOnIntegerOverflow=off  InputSameDT=off
  w01 : Constant  SampleTime=Ts_Control
  w1 : Constant  Commented=on  Value=2*pi*50  SampleTime=Ts_Control
  w2 : Constant  SampleTime=Ts_Control
  theta : Outport  VectorParamsAs1DForOutWhenUnconnected=off
  Vdref : Outport  Port=2
  wires:
  Sum4/1 -> theta/1
  Integrator2/1(Theta) -> Sum4/2
  w2/1 -> Integrator2/1(w)
  [delta_P] -> Integrator1/1(w)
  w01/1 -> Sum5/2
  passing flag2/1 -> Scope2/1, Sum1/1
  Sum/1 -> passing flag2/1, [delta_P]
  Transfer Fcn3/1 -> Sum5/1, Scope2/2, Integrator/1(w)
  Sum1/1 -> Transfer Fcn3/1
  Gain1/1 -> Sum1/2
  Sum5/1 -> Gain1/1
  fsys/1 -> Gain/1
  Constant2/1 -> passing flag2/3
  V_inv_mag/1 -> passing flag2/2
  Sum3/1 -> Scope9/1  "vdref"
  Reactive Controller/1 -> Sum3/1, Scope10/2
  Sum2/1 -> Reactive Controller/1, Scope10/1
  Demux1/2 -> Scope1/1, Sum2/2
  Demux/2 -> Scope6/1, Sum2/1  "Qref"
  Demux/1 -> Sum/1, Scope7/1  "Pref"
  PQref/1 -> Demux/1
  m/1 -> Demux1/1
  Demux1/1 -> Scope8/1, Sum/2
  Integrator/1(Theta) -> Scope3/1
  V0/1 -> Vdref/1
  Integrator1/1(Theta) -> Sum4/1

== system different_inverter_controls_BPS/GFM-VSG-100MW/FRT/In -RSY/PLL0/Moving Average1 ==
  In1 : Inport
  Ground1 : Ground
  Terminator1 : Terminator
  Out1 : Outport
  wires:
  Ground1/1 -> Out1/1
  In1/1 -> Terminator1/1

== system different_inverter_controls_BPS/GFM-VSG-100MW/FRT/In -RSY/PLL0/PI ==
  In1 : Inport
  Discrete-Time Integrator1 : DiscreteIntegrator  gainval=inv1.ki_pll/(2*pi*60)  SampleTime=Ts_Control  ICPrevOutput=DiscIntNeverNeededParam  ICPrevScaledInput=DiscIntNeverNeededParam
  Gain : Gain  Gain=inv1.kp_pll/(2*pi*60)
  Sum1 : Sum
  Out1 : Outport
  wires:
  In1/1 -> Discrete-Time Integrator1/1, Gain/1
  Gain/1 -> Sum1/1
  Discrete-Time Integrator1/1 -> Sum1/2
  Sum1/1 -> Out1/1

== system different_inverter_controls_BPS/GFM-VSG-100MW/FRT/In -RSY/PLL0/Subsystem ==
  In1 : Inport
  Constant4 : Constant  Value=0.0004999
  Constant5 : Constant  Value=-0.9998
  Constant6 : Constant  Value=0
  Discrete Varying Transfer Function : cstblocks/Linear Parameter Varying/Discrete Varying Transfer Function  N=1  Feedthrough=on  Ts=-1
  Out1 : Outport  VectorParamsAs1DForOutWhenUnconnected=off
  wires:
  Constant5/1 -> Discrete Varying Transfer Function/3
  Constant6/1 -> Discrete Varying Transfer Function/4
  Constant4/1 -> Discrete Varying Transfer Function/2
  Discrete Varying Transfer Function/1 -> Out1/1
  In1/1 -> Discrete Varying Transfer Function/1

== system different_inverter_controls_BPS/GFM-VSG-100MW/FRT/In -RSY/PLL3/Moving Average1 ==
  In1 : Inport
  Ground1 : Ground
  Terminator1 : Terminator
  Out1 : Outport
  wires:
  Ground1/1 -> Out1/1
  In1/1 -> Terminator1/1

== system different_inverter_controls_BPS/GFM-VSG-100MW/FRT/In -RSY/PLL3/PI ==
  In1 : Inport
  Discrete-Time Integrator1 : DiscreteIntegrator  gainval=inv1.ki_pll/(2*pi*60)  SampleTime=Ts_Control  ICPrevOutput=DiscIntNeverNeededParam  ICPrevScaledInput=DiscIntNeverNeededParam
  Gain : Gain  Gain=inv1.kp_pll/(2*pi*60)
  Sum1 : Sum
  Out1 : Outport
  wires:
  In1/1 -> Discrete-Time Integrator1/1, Gain/1
  Gain/1 -> Sum1/1
  Discrete-Time Integrator1/1 -> Sum1/2
  Sum1/1 -> Out1/1

== system different_inverter_controls_BPS/GFM-VSG-100MW/FRT/In -RSY/PLL3/Subsystem ==
  In1 : Inport
  Constant4 : Constant  Value=0.0004999
  Constant5 : Constant  Value=-0.9998
  Constant6 : Constant  Value=0
  Discrete Varying Transfer Function : cstblocks/Linear Parameter Varying/Discrete Varying Transfer Function  N=1  Feedthrough=on  Ts=-1
  Out1 : Outport  VectorParamsAs1DForOutWhenUnconnected=off
  wires:
  Constant5/1 -> Discrete Varying Transfer Function/3
  Constant6/1 -> Discrete Varying Transfer Function/4
  Constant4/1 -> Discrete Varying Transfer Function/2
  Discrete Varying Transfer Function/1 -> Out1/1
  In1/1 -> Discrete Varying Transfer Function/1

== system different_inverter_controls_BPS/GFM-VSG-100MW/FRT/In -RSY/Sync Check Control/PI1 ==
  In1 : Inport
  Discrete-Time Integrator1 : DiscreteIntegrator  gainval=ki_sync  SampleTime=Ts_Control  ICPrevOutput=DiscIntNeverNeededParam  ICPrevScaledInput=DiscIntNeverNeededParam
  Gain : Gain  Gain=kp_sync
  Sum1 : Sum
  Out1 : Outport
  wires:
  Discrete-Time Integrator1/1 -> Sum1/2
  In1/1 -> Discrete-Time Integrator1/1, Gain/1
  Gain/1 -> Sum1/1
  Sum1/1 -> Out1/1

== system different_inverter_controls_BPS/GFM-VSG-100MW/IBR-GFM VSG/Inverter/BESS Reference /Qref ==
  Constant : Constant  Value=44e6
  From1 : From  Commented=on  GotoTag=Q_BESS
  Out1 : Outport
  wires:
  Constant/1 -> Out1/1

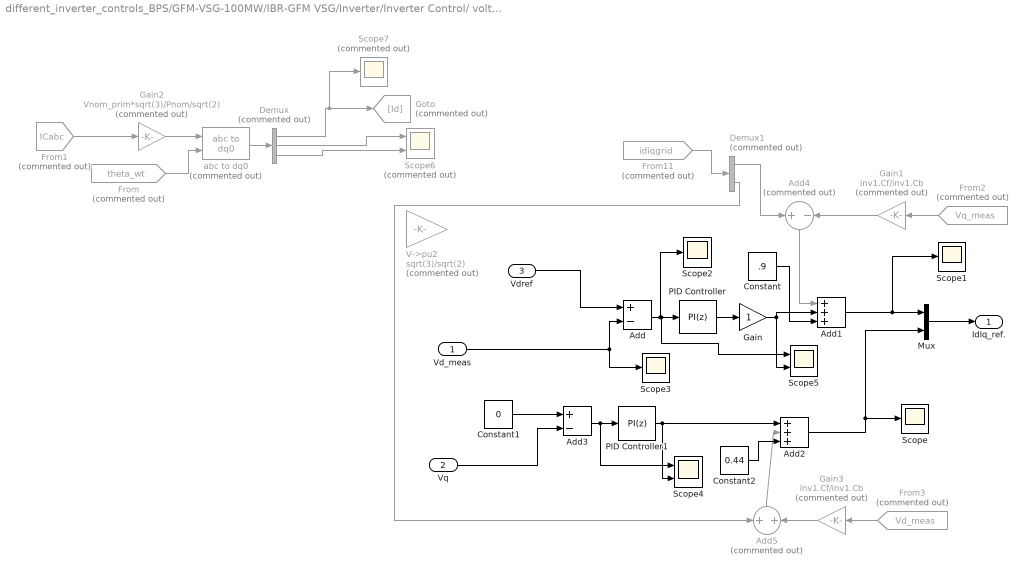
== system different_inverter_controls_BPS/GFM-VSG-100MW/IBR-GFM VSG/Inverter/Inverter Control/ voltage control  ==
  Vd_meas : Inport
  Vq : Inport  Port=2
  Vdref : Inport  Port=3
  Add : Sum  Inputs=+-
  Add1 : Sum  Inputs=+++
  Add2 : Sum  Inputs=+++
  Add3 : Sum  Inputs=+-
  Add4 : Sum  Commented=on  Inputs=+-
  Add5 : Sum  Commented=on
  Constant : Constant  Value=.9  SampleTime=Ts_Control
  Constant1 : Constant  Value=0
  Constant2 : Constant  Value=0.44
  Demux : Demux  Commented=on  Outputs=3
  Demux1 : Demux  Commented=on  Outputs=2
  From : From  Commented=on  GotoTag=theta_wt  TagVisibility=global
  From1 : From  Commented=on  GotoTag=ICabc  TagVisibility=global
  From11 : From  Commented=on  GotoTag=idiqgrid  TagVisibility=global
  From2 : From  Commented=on  GotoTag=Vq_meas  TagVisibility=global
  From3 : From  Commented=on  GotoTag=Vd_meas  TagVisibility=global
  Gain : Gain
  Gain1 : Gain  Commented=on  Gain=inv1.Cf/inv1.Cb
  Gain2 : Gain  Commented=on  Gain=Vnom_prim*sqrt(3)/Pnom/sqrt(2)
  Gain3 : Gain  Commented=on  Gain=inv1.Cf/inv1.Cb
  Goto : Goto  Commented=on  GotoTag=Id
  Mux : Mux  Inputs=2
  PID Controller : slpidlib/PID Controller  Controller=PI  Form=Parallel  TimeDomain=Discrete-time  UseExternalTs=off  SampleTime=Ts_Control  IntegratorMethod=Forward Euler  FilterMethod=Forward Euler  ControllerParametersSource=internal  P=.8  I=0  UseKiTs=off  D=0  UseExternalDerivativeSource=off  N=100  UseFilter=on  TunerSelectOption=Transfer Function Based (PID Tuner App)  InitialConditionSource=internal  InitialConditionForIntegrator=0  InitialConditionForFilter=0  DifferentiatorICPrevScaledInput=0  ExternalReset=none  TrackingMode=off  Kt=1  LimitOutput=on  SatLimitsSource=internal  UpperSaturationLimit=inf  LowerSaturationLimit=-inf  LinearizeAsGain=on  AntiWindupMode=back-calculation  Kb=1  LimitIntegrator=off  UpperIntegratorSaturationLimit=inf  LowerIntegratorSaturationLimit=-inf  POutMin=[]  POutMax=[]  IOutMin=[]  IOutMax=[]  DOutMin=[]  DOutMax=[]  NOutMin=[]  NOutMax=[]  SumOutMin=[]  SumOutMax=[]  SaturationOutMin=[]  SaturationOutMax=[]  PParamMin=[]  PParamMax=[]  IParamMin=[]  IParamMax=[]  DParamMin=[]  DParamMax=[]  NParamMin=[]  NParamMax=[]  KbParamMin=[]  KbParamMax=[]  KtParamMin=[]  KtParamMax=[]  KbOutMin=[]  KbOutMax=[]  KtOutMin=[]  KtOutMax=[]  IntegratorOutMin=[]  IntegratorOutMax=[]  FilterOutMin=[]  FilterOutMax=[]  SumI1OutMin=[]  SumI1OutMax=[]  SumI2OutMin=[]  SumI2OutMax=[]  SumI3OutMin=[]  SumI3OutMax=[]  SumI4OutMin=[]  SumI4OutMax=[]  SumDOutMin=[]  SumDOutMax=[]  DifferentiatorOutMin=[]  DifferentiatorOutMax=[]  FilterDiffOutCoefMin=[]  FilterDiffOutCoefMax=[]  ReciprocalOutMin=[]  ReciprocalOutMax=[]  SumDenOutMin=[]  SumDenOutMax=[]  SumNumOutMin=[]  SumNumOutMax=[]  DivideOutMin=[]  DivideOutMax=[]  UdiffTsProdOutMin=[]  UdiffTsProdOutMax=[]  NTsProdOutMin=[]  NTsProdOutMax=[]  UintegralTsProdOutMin=[]  UintegralTsProdOutMax=[]  UngainTsProdOutMin=[]  UngainTsProdOutMax=[]  ClampingZeroOutDataTypeStr=Inherit: Inherit via back propagation  ClampingZeroOutMin=[]  ClampingZeroOutMax=[]  FilterDenConstantOutDataTypeStr=Inherit: Inherit via back propagation  FilterDenConstantOutMin=[]  FilterDenConstantOutMax=[]  PCopyOutDataTypeStr=Inherit: Inherit via back propagation  PCopyOutMin=[]  PCopyOutMax=[]  NCopyOutDataTypeStr=Inherit: Inherit via back propagation  NCopyOutMin=[]  NCopyOutMax=[]  IntegratorContinuousStateAttributes=''  IntegratorStateMustResolveToSignalObject=off  IntegratorRTWStateStorageClass=Auto  FilterContinuousStateAttributes=''  FilterStateMustResolveToSignalObject=off  FilterRTWStateStorageClass=Auto  ParallelPVariant=InternalParameters  IdealPVariant=Disabled  IVariant=InternalParameters  DVariant=Disabled  IntegratorVariant=Discrete  SatVariant=Enabled  AWVariant=BackCalculation  PCopyVariant=Disabled  TRVariant=Disabled  FdbkBlocksVariant=Forward  IdealPFdbkVariant=Disabled  SatFdbkVariant=Disabled  DerivativeFilterVariant=Disabled  NVariant=Disabled  NCopyVariant=Disabled_SignalSpec  FilterICVariant=Disabled  IntegratorICVariant=InternalICs  ExternalResetVariant=Disabled  TRSumVariant=Passthrough  SumFdbkVariant=Disabled  SumVariant=Sum_PI  TsampFilterVariant=InternalTs  TsampNgainVariant=Passthrough  TsampIntegralVariant=Disabled_SignalSpec  ExternalSaturationOutDataTypeStr=Inherit: Same as second input  DerivativeSourceVariant=Disabled  PreIntVariant=InternalPreInt
  PID Controller1 : slpidlib/PID Controller  Controller=PI  Form=Parallel  TimeDomain=Discrete-time  UseExternalTs=off  SampleTime=Ts_Control  IntegratorMethod=Forward Euler  FilterMethod=Forward Euler  ControllerParametersSource=internal  P=.79  I=0  UseKiTs=off  D=0  UseExternalDerivativeSource=off  N=100  UseFilter=on  TunerSelectOption=Transfer Function Based (PID Tuner App)  InitialConditionSource=internal  InitialConditionForIntegrator=0  InitialConditionForFilter=0  DifferentiatorICPrevScaledInput=0  ExternalReset=none  TrackingMode=off  Kt=1  LimitOutput=on  SatLimitsSource=internal  UpperSaturationLimit=inf  LowerSaturationLimit=-inf  LinearizeAsGain=on  AntiWindupMode=back-calculation  Kb=1  LimitIntegrator=off  UpperIntegratorSaturationLimit=inf  LowerIntegratorSaturationLimit=-inf  POutMin=[]  POutMax=[]  IOutMin=[]  IOutMax=[]  DOutMin=[]  DOutMax=[]  NOutMin=[]  NOutMax=[]  SumOutMin=[]  SumOutMax=[]  SaturationOutMin=[]  SaturationOutMax=[]  PParamMin=[]  PParamMax=[]  IParamMin=[]  IParamMax=[]  DParamMin=[]  DParamMax=[]  NParamMin=[]  NParamMax=[]  KbParamMin=[]  KbParamMax=[]  KtParamMin=[]  KtParamMax=[]  KbOutMin=[]  KbOutMax=[]  KtOutMin=[]  KtOutMax=[]  IntegratorOutMin=[]  IntegratorOutMax=[]  FilterOutMin=[]  FilterOutMax=[]  SumI1OutMin=[]  SumI1OutMax=[]  SumI2OutMin=[]  SumI2OutMax=[]  SumI3OutMin=[]  SumI3OutMax=[]  SumI4OutMin=[]  SumI4OutMax=[]  SumDOutMin=[]  SumDOutMax=[]  DifferentiatorOutMin=[]  DifferentiatorOutMax=[]  FilterDiffOutCoefMin=[]  FilterDiffOutCoefMax=[]  ReciprocalOutMin=[]  ReciprocalOutMax=[]  SumDenOutMin=[]  SumDenOutMax=[]  SumNumOutMin=[]  SumNumOutMax=[]  DivideOutMin=[]  DivideOutMax=[]  UdiffTsProdOutMin=[]  UdiffTsProdOutMax=[]  NTsProdOutMin=[]  NTsProdOutMax=[]  UintegralTsProdOutMin=[]  UintegralTsProdOutMax=[]  UngainTsProdOutMin=[]  UngainTsProdOutMax=[]  ClampingZeroOutDataTypeStr=Inherit: Inherit via back propagation  ClampingZeroOutMin=[]  ClampingZeroOutMax=[]  FilterDenConstantOutDataTypeStr=Inherit: Inherit via back propagation  FilterDenConstantOutMin=[]  FilterDenConstantOutMax=[]  PCopyOutDataTypeStr=Inherit: Inherit via back propagation  PCopyOutMin=[]  PCopyOutMax=[]  NCopyOutDataTypeStr=Inherit: Inherit via back propagation  NCopyOutMin=[]  NCopyOutMax=[]  IntegratorContinuousStateAttributes=''  IntegratorStateMustResolveToSignalObject=off  IntegratorRTWStateStorageClass=Auto  FilterContinuousStateAttributes=''  FilterStateMustResolveToSignalObject=off  FilterRTWStateStorageClass=Auto  ParallelPVariant=InternalParameters  IdealPVariant=Disabled  IVariant=InternalParameters  DVariant=Disabled  IntegratorVariant=Discrete  SatVariant=Enabled  AWVariant=BackCalculation  PCopyVariant=Disabled  TRVariant=Disabled  FdbkBlocksVariant=Forward  IdealPFdbkVariant=Disabled  SatFdbkVariant=Disabled  DerivativeFilterVariant=Disabled  NVariant=Disabled  NCopyVariant=Disabled_SignalSpec  FilterICVariant=Disabled  IntegratorICVariant=InternalICs  ExternalResetVariant=Disabled  TRSumVariant=Passthrough  SumFdbkVariant=Disabled  SumVariant=Sum_PI  TsampFilterVariant=InternalTs  TsampNgainVariant=Passthrough  TsampIntegralVariant=Disabled_SignalSpec  ExternalSaturationOutDataTypeStr=Inherit: Same as second input  DerivativeSourceVariant=Disabled  PreIntVariant=InternalPreInt
  Scope{,1..3} (4 alike) : Scope
  Scope4 : Scope  NumInputPorts=2
  Scope5 : Scope  NumInputPorts=2
  Scope6 : Scope  Commented=on  NumInputPorts=2
  Scope7 : Scope  Commented=on
  V->pu2 : Gain  Commented=on  Gain=sqrt(3)/sqrt(2)  SaturateOnIntegerOverflow=on  OutDataTypeStr=Inherit: Same as input  ParamDataTypeStr=Inherit: Same as input
  abc to dq0 : spsabctodq0Lib/abc to dq0  Commented=on  Alignment=90 degrees behind phase A axis
  IdIq_ref. : Outport
  wires:
  Demux/3 -> Scope6/2
  Demux/2 -> Scope6/1
  Demux/1 -> Goto/1, Scope7/1
  abc to dq0/1 -> Demux/1
  From1/1 -> Gain2/1
  Gain2/1 -> abc to dq0/1
  From/1 -> abc to dq0/2
  Add2/1 -> Mux/2, Scope/1
  PID Controller1/1 -> Add2/1, Scope4/2
  Add1/1 -> Mux/1, Scope1/1
  Gain/1 -> Add1/2, Scope5/2
  Mux/1 -> IdIq_ref./1
  Add/1 -> Scope5/1, PID Controller/1, Scope2/1
  PID Controller/1 -> Gain/1
  Vd_meas/1 -> Scope3/1, Add/2
  Vdref/1 -> Add/1
  Constant1/1 -> Add3/1
  Vq/1 -> Add3/2
  Add3/1 -> Scope4/1, PID Controller1/1
  Add4/1 -> Add1/1
  From11/1 -> Demux1/1
  Demux1/1 -> Add4/1
  Gain1/1 -> Add4/2
  From2/1 -> Gain1/1
  Demux1/2 -> Add5/1
  Add5/1 -> Add2/2
  Gain3/1 -> Add5/2
  From3/1 -> Gain3/1
  Constant/1 -> Add1/3
  Constant2/1 -> Add2/3

== system different_inverter_controls_BPS/GFM-VSG-100MW/IBR-GFM VSG/Inverter/Inverter Control/Conversions ==
  Vabc_prim : Inport
  Iabc_prim : Inport  Port=2
  Iabc_grid : Inport  Port=3
  From1 : From  Commented=on  GotoTag=theta_inv  TagVisibility=global
  From2 : From  Commented=on  GotoTag=theta  TagVisibility=global
  Goto7 : Goto  Commented=on  GotoTag=theta_inv  TagVisibility=global
  PLL (3ph)1 : spsPLL3phLib/PLL (3ph)  Fmin=45  Par_Init="[-0.57  Fnom]"  ParK=[180, 3200, 1]  TcD=1e-04  MaxRateChangeFreq=12  FilterCutOffFreq=25  Ts=Ts_Control  AGC=on
      link override Model/Constant4: Value=2*pi
  "PMU (PLL-Based, Positive-Sequence)" : spsPMUPLLBasedPositiveSequenceLib/PMU (PLL-Based, Positive-Sequence)  Commented=on  nominalFrequency=50  samplingRate=64  reportingFactor=1
  Scope{,1..3,7} (5 alike) : Scope
  Scope4 : Scope  Commented=on
  Scope5 : Scope  Commented=on
  Scope6 : Scope  Commented=on
  Selector1 : Selector  InputPortWidth=3  IndexOptions=Index vector (dialog)  Indices=[1 2]  OutputSizes=1
  Selector2 : Selector  InputPortWidth=3  IndexOptions=Index vector (dialog)  Indices=[1 2]  OutputSizes=1
  Selector3 : Selector  Commented=on  InputPortWidth=3  IndexOptions=Index vector (dialog)  Indices=[1 2]  OutputSizes=1
  Terminator : Terminator  Commented=on
  Terminator1 : Terminator  Commented=on
  V->pu : Gain  Gain=1/(Vpp*sqrt(2)/sqrt(3))  SaturateOnIntegerOverflow=on  OutDataTypeStr=Inherit: Same as input  ParamDataTypeStr=Inherit: Same as input
  V->pu1 : Gain  Gain=Vpp*sqrt(3)/Pnom/sqrt(2)  SaturateOnIntegerOverflow=on  OutDataTypeStr=Inherit: Same as input  ParamDataTypeStr=Inherit: Same as input
  V->pu2 : Gain  Commented=on  Gain=1/(Vnom_prim*sqrt(2)/sqrt(3))  SaturateOnIntegerOverflow=on  OutDataTypeStr=Inherit: Same as input  ParamDataTypeStr=Inherit: Same as input
  V->pu3 : Gain  Commented=on  Gain=Vnom_prim*sqrt(3)/Pnom/sqrt(2)  SaturateOnIntegerOverflow=on  OutDataTypeStr=Inherit: Same as input  ParamDataTypeStr=Inherit: Same as input
  V->pu4 : Gain  Commented=on  Gain=1/(Vpp*sqrt(2)/sqrt(3))  SaturateOnIntegerOverflow=on  OutDataTypeStr=Inherit: Same as input  ParamDataTypeStr=Inherit: Same as input
  V->pu6 : Gain  Commented=on  Gain=Vnom_prim*sqrt(3)/Pnom/sqrt(2)  SaturateOnIntegerOverflow=on  OutDataTypeStr=Inherit: Same as input  ParamDataTypeStr=Inherit: Same as input
  abc to dq0 : spsabctodq0Lib/abc to dq0  Alignment=90 degrees behind phase A axis
  abc to dq1 : spsabctodq0Lib/abc to dq0  Alignment=90 degrees behind phase A axis
  abc to dq2 : spsabctodq0Lib/abc to dq0  Commented=on  Alignment=90 degrees behind phase A axis
  wt : Outport  VectorParamsAs1DForOutWhenUnconnected=off
  VdVq_prim : Outport  Port=2  VectorParamsAs1DForOutWhenUnconnected=off
  IdIq_prim : Outport  Port=3  VectorParamsAs1DForOutWhenUnconnected=off
  IdIq_grid : Outport  Port=4  VectorParamsAs1DForOutWhenUnconnected=off
  tag scope: PLL_Freq=scoped, theta_wt=global
  wires:
  V->pu1/1 -> abc to dq1/1, Scope1/1
  PLL (3ph)1/2 -> Scope/1, [theta_wt], wt/1
  Selector1/1 -> IdIq_prim/1, Scope2/1
  Selector2/1 -> VdVq_prim/1
  abc to dq0/1 -> Selector2/1
  Iabc_prim/1 -> V->pu1/1
  Vabc_prim/1 -> V->pu/1
  abc to dq1/1 -> Selector1/1
  V->pu/1 -> "PMU (PLL-Based, Positive-Sequence)"/1, PLL (3ph)1/1, Scope7/1, abc to dq0/1
  PLL (3ph)1/1 -> Scope3/1, [PLL_Freq]
  "PMU (PLL-Based, Positive-Sequence)"/2 -> Scope4/1, Goto7/1
  "PMU (PLL-Based, Positive-Sequence)"/3 -> Terminator/1
  "PMU (PLL-Based, Positive-Sequence)"/1 -> Terminator1/1
  [theta] -> abc to dq0/2, abc to dq2/2, abc to dq1/2
  abc to dq2/1 -> Selector3/1
  Selector3/1 -> Scope6/1, IdIq_grid/1
  Iabc_grid/1 -> Scope5/1, abc to dq2/1

== system different_inverter_controls_BPS/GFM-VSG-100MW/IBR-GFM VSG/Inverter/Inverter Control/Current Control ==
  wt : Inport
  VdVq_meas : Inport  Port=2  PortDimensions=2
  IdIq_meas : Inport  Port=3  PortDimensions=2
  IdIq_ref : Inport  Port=4  PortDimensions=2
  Current Regulator : Subsystem
  Uabc_ref Generation max (m) = 1 : Subsystem
  Uabc : Outport  VectorParamsAs1DForOutWhenUnconnected=off
  wires:
  wt/1 -> Uabc_ref Generation max (m) = 1/1(wt)
  Current Regulator/1(VdVq_conv) -> Uabc_ref Generation max (m) = 1/2(VdVq_conv)
  VdVq_meas/1 -> Current Regulator/1(VdVq_meas)
  IdIq_meas/1 -> Current Regulator/2(IdIq_meas)
  IdIq_ref/1 -> Current Regulator/3(IdIq_ref)
  Uabc_ref Generation max (m) = 1/1(Uabc_ref) -> Uabc/1

== system different_inverter_controls_BPS/GFM-VSG-100MW/IBR-GFM VSG/Inverter/Inverter Control/current limiter ==
  note: P or Q priority limits are usually applied during grid feeding mode of operation
      | https://www.esig.energy/wiki-main-page/wecc-distributed-and-small-pv-plants-generic-model-pvd1/
  idiqPref : Inport
  V_inv_mag : Inport  Port=2
  P priority limit : Subsystem  Commented=on
  Q priority limit : Subsystem
  Subsystem3 : Subsystem  Commented=on
  Subsystem4 : Subsystem  Commented=on
  Subsystem9 : Subsystem
  Switch1 : Switch  Commented=on  Criteria=u2 > Threshold  SaturateOnIntegerOverflow=off  InputSameDT=off
  idiqPRefL : Outport
  wires:
  Subsystem3/2(Out2) -> [IPvector]
  [Ivector] -> Subsystem9/1(In1)
  Subsystem4/1(Out1) -> Switch1/1
  [Ivector] -> Subsystem4/1(In1)
  Subsystem3/1(Out1) -> [Ivector]
  idiqPref/1 -> Subsystem3/1(In1), P priority limit/1(idiqP), Q priority limit/1(idiqP), Subsystem9/2(In2), Subsystem4/2(In2)
  Q priority limit/1(idiqPRefL) -> idiqPRefL/1, Switch1/3
  [mode] -> Switch1/2
  V_inv_mag/1 -> Q priority limit/2(V_inv_mag)

== system different_inverter_controls_BPS/GFM-VSG-100MW/IBR-GFM VSG/Inverter/Power Controller/Compute PQ ==
  m : Inport
  Bus Selector : BusSelector  OutputSignals=Vabc,Iabc
  Mux : Mux  Inputs=2
  "Power (3ph, Instantaneous)" : spsPower3phInstantaneousLib/Power (3ph, Instantaneous)
  Scope1 : Scope
  to PU : Gain  Gain=1/Pnom
  "to PU " : Gain  Gain=1/Pnom
  to PU1 : Gain  Commented=on  Gain=1/Pnom
  PQm : Outport  VectorParamsAs1DForOutWhenUnconnected=off
  wires:
  Mux/1 -> Scope1/1, PQm/1
  "to PU "/1 -> Mux/2
  to PU/1 -> Mux/1
  m/1 -> Bus Selector/1
  "Power (3ph, Instantaneous)"/1 -> to PU/1
  Bus Selector/2 -> "Power (3ph, Instantaneous)"/2  "<Iabc>"
  "Power (3ph, Instantaneous)"/2 -> "to PU "/1
  Bus Selector/1 -> "Power (3ph, Instantaneous)"/1  "<Vabc>"
